simulink model "TestAssignmentImplementingChannelComms"  (R2017b)
settings: Solver=FixedStepAuto  StartTime=0.0  StopTime=100  FixedStep=1  RelTol=1e-3
undefined symbols (not defined in the file): ok
settings Model: Creator=georgimarkov  LastModifiedBy=georgimarkov

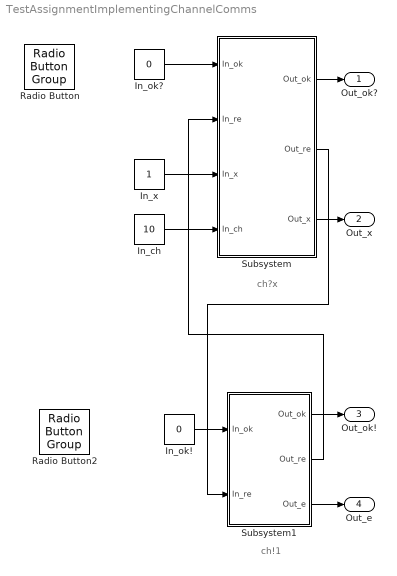
== system TestAssignmentImplementingChannelComms ==
  note: ch?x
  note: ch!1
  In_ch : Constant  Value=10
  In_ok! : Constant  Value=0
  In_ok? : Constant  Value=0
  In_x : Constant
  Radio Button : RadioButtonGroup  WebBlockId=28  ModelName=TestAssignmentImplementingChannelComms  LabelPosition=Top  ShowInitialText=on  SelectedLabel=-ok  ButtonGroupName=Group
      settings: Values={{'-ok', 'ok'}, [0 1]}
  Radio Button2 : RadioButtonGroup  WebBlockId=60  ModelName=TestAssignmentImplementingChannelComms  LabelPosition=Top  ShowInitialText=on  SelectedLabel=-ok  ButtonGroupName=Group
      settings: Values={{'-ok', 'ok'}, [0 1]}
  Subsystem : Subsystem
  Subsystem1 : Subsystem
  Out_ok? : Outport
  "Out_x " : Outport  Port=2
  Out_ok! : Outport  Port=3
  Out_e : Outport  Port=4
  wires:
  In_ok?/1 -> Subsystem/1(In_ok)
  Subsystem1/2(Out_re) -> Subsystem/2(In_re)
  In_x/1 -> Subsystem/3("In_x ")
  In_ch/1 -> Subsystem/4(In_ch)
  Subsystem/1(Out_ok) -> Out_ok?/1
  Subsystem/3("Out_x ") -> "Out_x "/1
  In_ok!/1 -> Subsystem1/1(In_ok)
  Subsystem/2(Out_re) -> Subsystem1/2(In_re)
  Subsystem1/1(Out_ok) -> Out_ok!/1
  Subsystem1/3(Out_e) -> Out_e/1

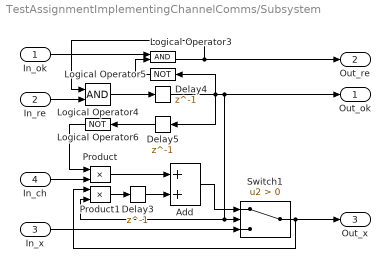
== system TestAssignmentImplementingChannelComms/Subsystem ==
  In_ok : Inport
  In_re : Inport  Port=2
  "In_x " : Inport  Port=3
  In_ch : Inport  Port=4
  Add : Sum
  Delay3 : Delay  DelayLength=1  InitialCondition=0
  Delay4 : Delay  DelayLength=1  InitialCondition=0
  Delay5 : Delay  DelayLength=1  InitialCondition=0
  Logical Operator3 : Logic  AllPortsSameDT=off  OutDataTypeStr=fixdt(1,16)
  Logical Operator4 : Logic  AllPortsSameDT=off  OutDataTypeStr=fixdt(1,16)
  Logical Operator5 : Logic  Operator=NOT  AllPortsSameDT=off  OutDataTypeStr=fixdt(1,16)
  Logical Operator6 : Logic  Operator=NOT  AllPortsSameDT=off  OutDataTypeStr=fixdt(1,16)
  Product : Product
  Product1 : Product
  Switch1 : Switch  Criteria=u2 > Threshold
  Out_ok : Outport
  Out_re : Outport  Port=2
  "Out_x " : Outport  Port=3
  wires:
  Delay5/1 -> Logical Operator6/1
  In_ok/1 -> Logical Operator3/1
  Product1/1 -> Delay3/1
  Logical Operator4/1 -> Delay4/1
  Switch1/1 -> "Out_x "/1, Product1/1
  "In_x "/1 -> Switch1/3
  In_re/1 -> Logical Operator4/2
  Product/1 -> Add/1
  Delay3/1 -> Add/2
  In_ch/1 -> Product/2
  Delay4/1 -> Delay5/1, Logical Operator5/1, Out_ok/1, Product1/2, Switch1/2
  Logical Operator5/1 -> Logical Operator3/2
  Logical Operator3/1 -> Out_re/1, Logical Operator4/1
  Logical Operator6/1 -> Product/1
  Add/1 -> Switch1/1

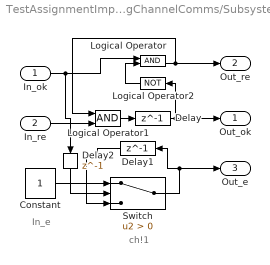
== system TestAssignmentImplementingChannelComms/Subsystem1 ==
  note: ch!1
  note: In_e
  In_ok : Inport
  In_re : Inport  Port=2
  Constant : Constant
  Delay : Delay  DelayLength=1  InitialCondition=0
  Delay1 : Delay  DelayLength=1  InitialCondition=0
  Delay2 : Delay  DelayLength=1  InitialCondition=0
  Logical Operator : Logic  AllPortsSameDT=off  OutDataTypeStr=fixdt(1,16)
  Logical Operator1 : Logic  AllPortsSameDT=off  OutDataTypeStr=fixdt(1,16)
  Logical Operator2 : Logic  Operator=NOT  AllPortsSameDT=off  OutDataTypeStr=boolean
  Switch : Switch  Criteria=u2 > Threshold
  Out_ok : Outport
  Out_re : Outport  Port=2
  Out_e : Outport  Port=3
  wires:
  In_re/1 -> Logical Operator1/2
  Delay1/1 -> Switch/3
  Switch/1 -> Out_e/1, Delay1/1
  In_ok/1 -> Logical Operator/1, Delay2/1
  Delay2/1 -> Switch/2
  Delay/1 -> Out_ok/1, Logical Operator2/1
  Logical Operator1/1 -> Delay/1
  Constant/1 -> Switch/1
  Logical Operator/1 -> Out_re/1, Logical Operator1/1
  Logical Operator2/1 -> Logical Operator/2
